simulink model "example"  (R2022b)
settings: Solver=VariableStepAuto  StartTime=0.0  StopTime=10.0  RelTol=1e-3
undefined symbols (not defined in the file): Discrete, Time
libraries: ctrlSharedLib x1
settings Model: Creator=saigon  LastModifiedBy=saigon
settings DebuggingCC: UnconnectedInputMsg=warning  UnconnectedOutputMsg=warning  UnconnectedLineMsg=warning
settings ModelReferenceCC: EnableRefExpFcnMdlSchedulingChecks=on
settings RTWCC: DLArmComputeVersion=19.05

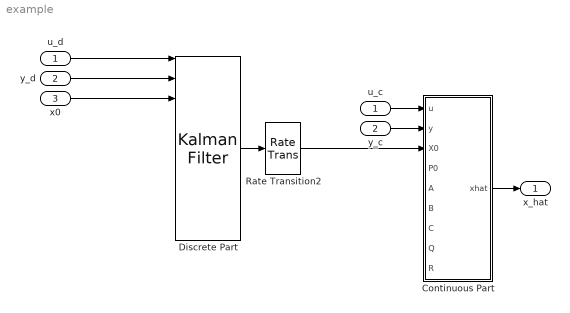
== system example ==
  u_d : Inport
  y_c : Inport  Port=2
  x0 : Inport  Port=3
  Continuous Part : Subsystem
  Discrete Part : ctrlSharedLib/Kalman Filter  TimeDomain=Discrete-Time  UseCurrentEstimator=on  ModelSource=Input port  ModelSourceVariable=ss(0.95,1,1,0,1)  A=0.95  B=1  C=1  D=0  NumberOfStates=1  NumberOfInputs=1  NumberOfOutputs=1  InitialEstimateSource=Input port  X0=0  P0=10  UseK=off  UseGH=off  NumberOfProcessNoiseInputs=1  G=1  TimeInvariantG=on  H=0  TimeInvariantH=on  Q=0.05  TimeInvariantQ=off  R=1  TimeInvariantR=off  N=0  TimeInvariantN=on  AddInputPort=on  AddEnablePort=off  OutputEstimatedY=off  OutputP=off  Ts=-1
  Rate Transition2 : RateTransition
  u_c : InportShadow
  y_d : InportShadow  Port=2
  x_hat : Outport
  wires:
  Discrete Part/1 -> Rate Transition2/1
  Rate Transition2/1 -> Continuous Part/3(X0)
  u_d/1 -> Discrete Part/1
  u_c/1 -> Continuous Part/1(u)
  y_c/1 -> Continuous Part/2(y)
  y_d/1 -> Discrete Part/2
  x0/1 -> Discrete Part/3
  Continuous Part/1(xhat) -> x_hat/1
  ? -> Continuous Part/4(P0)
  ? -> Continuous Part/5(A)
  ? -> Continuous Part/6(B)
  ? -> Continuous Part/7(C)
  ? -> Continuous Part/8(Q)
  ? -> Continuous Part/9(R)
  ? -> Discrete Part/10
  ? -> Discrete Part/9
  ? -> Discrete Part/8
  ? -> Discrete Part/7
  ? -> Discrete Part/6
  ? -> Discrete Part/5
  ? -> Discrete Part/4

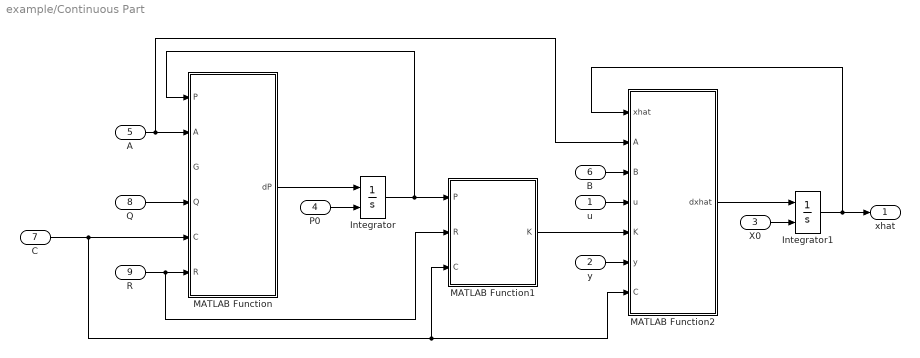
== system example/Continuous Part ==
  u : Inport
  y : Inport  Port=2
  X0 : Inport  Port=3
  P0 : Inport  Port=4
  A : Inport  Port=5
  B : Inport  Port=6
  C : Inport  Port=7
  Q : Inport  Port=8
  R : Inport  Port=9
  Integrator : Integrator  InitialConditionSource=external
  Integrator1 : Integrator  InitialConditionSource=external
  MATLAB Function : MATLAB Function  TreatAsAtomicUnit=on
  MATLAB Function1 : MATLAB Function  TreatAsAtomicUnit=on
  MATLAB Function2 : MATLAB Function  TreatAsAtomicUnit=on
  xhat : Outport
  wires:
  P0/1 -> Integrator/2
  y/1 -> MATLAB Function2/6(y)
  u/1 -> MATLAB Function2/4(u)
  B/1 -> MATLAB Function2/3(B)
  Integrator1/1 -> xhat/1, MATLAB Function2/1(xhat)
  MATLAB Function1/1(K) -> MATLAB Function2/5(K)
  X0/1 -> Integrator1/2
  MATLAB Function2/1(dxhat) -> Integrator1/1
  C/1 -> MATLAB Function/5(C), MATLAB Function1/3(C), MATLAB Function2/7(C)
  R/1 -> MATLAB Function/6(R), MATLAB Function1/2(R)
  Q/1 -> MATLAB Function/4(Q)
  A/1 -> MATLAB Function/2(A), MATLAB Function2/2(A)
  Integrator/1 -> MATLAB Function/1(P), MATLAB Function1/1(P)
  MATLAB Function/1(dP) -> Integrator/1

== matlab function example/Continuous Part/MATLAB Function ==
  data: P input; A input; dP output; G input; Q input; C input; R input
function dP = DerivativeP(P,A,G,Q,C,R)
G = eye(length(Q));
dP = A*P + P*A' + G*Q*G' - P*C'*inv(R)*C*P;

== matlab function example/Continuous Part/MATLAB Function1 ==
  data: P input; R input; K output; C input
function K = FilterGain(P,R,C)
K = P*C'*inv(R);

== matlab function example/Continuous Part/MATLAB Function2 ==
  data: xhat input; A input; B input; dxhat output; u input; K input; y input size=12; C input
function dxhat = DerivativeXHAT(xhat, A, B, u, K, y, C)
dxhat = A*xhat + B*u + K*(y - C*xhat);
